simulink model "ver_602"  (R2015b)
settings: Solver=FixedStepDiscrete  StartTime=0.0  StopTime=inf  FixedStep=0.1  RelTol=1e-3
StartFcn:
  | %The GUI handles are by default hidden, turn them on
  | set(0,'ShowHiddenHandles','on');
  | 
  | %Set up the arguments that will go into the gain block event callback listener
  | blk = 'ver_601/Clock';
  | event = 'PostOutputs';
  | listener = @up_gui_ver_301;
  | 
  | %Create the listener
  | h = add_exec_event_listener(blk, event, listener);
settings Model: PauseTimes=26500  NumberOfSteps=10  Creator=Ridvan  LastModifiedBy=Edmem10

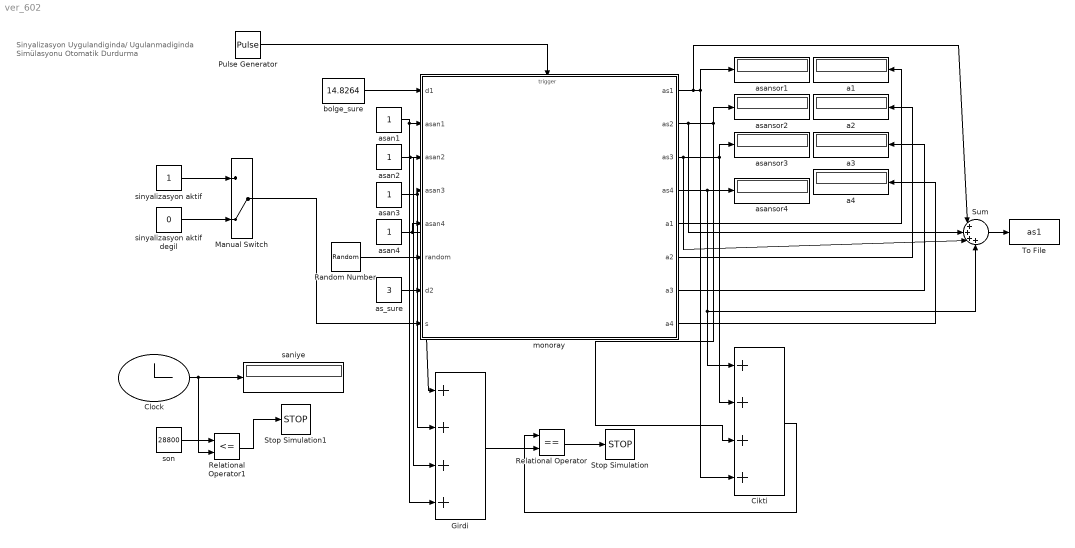
== system ver_602 ==
  note: Sinyalizasyon Uygulandiginda/ Ugulanmadiginda Simülasyonu Otomatik Durdurma
  Cikti : Sum  Inputs=++++
  Clock : Clock
      settings: Decimation=4
  Girdi : Sum  Inputs=++++
  Manual Switch : ManualSwitch  CurrentSetting=0
  Pulse Generator : DiscretePulseGenerator  PulseType=Time based  Period=1  PulseWidth=50
  Random Number : UniformRandomNumber  Minimum=0  Maximum=100  SampleTime=0.1
  Relational Operator : RelationalOperator  Operator===  OutDataTypeStr=boolean
  Relational Operator1 : RelationalOperator  Operator=<=  OutDataTypeStr=boolean
  Stop Simulation : Stop
  Stop Simulation1 : Stop
  Sum : Sum  Inputs=|++++
  To File : ToFile  Filename=as1  MatrixName=as1
  a{1..4} (4 alike) : Display
  as_sure : Constant  Value=3
  asan{1..4} (4 alike) : Constant
  asansor{1..4} (4 alike) : Display
  bolge_sure : Constant  Value=14.8264
  monoray : Stateflow chart  RequirementInfo="{}  %GIDa_5e52e2eb_da7a_4365_b597_b620b12073ae"  TreatAsAtomicUnit=on
  saniye : Display
  sinyalizasyon aktif : Constant
  sinyalizasyon aktif degil : Constant  Value=0
  son : Constant  Value=28800
  wires:
  Pulse Generator/1 -> monoray/Trigger
  monoray/2(as2) -> Sum/2, Cikti/3, asansor2/1
  monoray/1(as1) -> Sum/1, Cikti/4, asansor1/1
  monoray/3(as3) -> Sum/3, Cikti/2, asansor3/1
  bolge_sure/1 -> monoray/1(d1)
  Random Number/1 -> monoray/6(random)
  asan1/1 -> Girdi/4, monoray/2(asan1)
  asan2/1 -> Girdi/3, monoray/3(asan2)
  asan3/1 -> monoray/4(asan3), Girdi/2
  asan4/1 -> Girdi/1, monoray/5(asan4)
  as_sure/1 -> monoray/7(d2)
  monoray/5(a1) -> a1/1
  monoray/6(a2) -> a2/1
  monoray/7(a3) -> a3/1
  monoray/8(a4) -> a4/1
  Manual Switch/1 -> monoray/8(s)
  sinyalizasyon aktif/1 -> Manual Switch/1
  sinyalizasyon aktif degil/1 -> Manual Switch/2
  Clock/1 -> Relational Operator1/2, saniye/1
  Cikti/1 -> Relational Operator/1
  Girdi/1 -> Relational Operator/2
  Relational Operator/1 -> Stop Simulation/1
  Relational Operator1/1 -> Stop Simulation1/1
  son/1 -> Relational Operator1/1
  monoray/4(as4) -> Sum/4, Cikti/1, asansor4/1
  Sum/1 -> To File/1

== stateflow chart ver_602/monoray ==
  state m3
    state m1 [parallel]
      settings: executionOrder=1
      state r4 [parallel]
        settings: executionOrder=4
        state On
          en:vr4=1;
        state Next
          entry: vr5=1;
          dp5=dp4;
          vn5=vn4;
          vs5=vs4;
        state as1
          entry: as1 = as1 + 1;
          exit:dp4=0;
          vs4=0;
        state Off
          entry: vr4=0;
          dp4=0;
          vs4=0;
          vn4=0;
        m3.m1.r4.On -> m3.m1.r4.Next [order 2] : [after(d1, sec) & dp4~=1]
        m3.m1.r4.Off -> m3.m1.r4.On : [vr4==1]
        m3.m1.r4.On -> as1 [order 1] : [dp4==1 & after(d2,sec)]
        m3.m1.r4.Next -> m3.m1.r4.Off
        as1 -> m3.m1.r4.Next : [after(d1,sec)]{dp4=0;vs4=0;}
        (default) -> m3.m1.r4.Off
      state r5 [parallel]
        settings: executionOrder=5
        state On
          en:vr5=1;
        state Next1
          entry: vr6=1;
          dp6=dp5;
          vn6=vn5;
          vs6=vs5;
        state Next2
          entry: vr18=1;
          dp18=dp5;
          vn18=vn5;
          vs18=vs5;
        state Off
          entry: vr5=0;
          dp5=0;
          vs5=0;
          vn5=0;
        m3.m1.r5.On -> Next1 [order 2] : [after(d1, sec) & vr6==0]
        m3.m1.r5.On -> Next2 [order 1] : [(dp5==4 | dp5==0) & after(d1,sec) & vr18==0 & s==1]
        m3.m1.r5.Off -> m3.m1.r5.On : [vr5==1]
        Next1 -> m3.m1.r5.Off
        Next2 -> m3.m1.r5.Off
        (default) -> m3.m1.r5.Off
      state r8 [parallel]
        settings: executionOrder=8
        state On
          en:vr8=1;
        state Next
          entry: vr9=1;
          dp9=dp8;
          vn9=vn8;
          vs9=vs8;
        state Off
          entry: vr8=0;
          dp8=0;
          vs8=0;
          vn8=0;
        m3.m1.r8.On -> m3.m1.r8.Next : [after(d1, sec) & vr9==0]
        m3.m1.r8.Off -> m3.m1.r8.On : [vr8==1]
        m3.m1.r8.Next -> m3.m1.r8.Off
        (default) -> m3.m1.r8.Off
      state r9 [parallel]
        settings: executionOrder=9
        state On
          en:vr9=1;
        state Next
          entry: vr21=1;
          dp21=dp9;
          vn21=vn9;
          vs21=vs9;
        state Off
          entry: vr9=0;
          dp9=0;
          vs9=0;
          vn9=0;
        m3.m1.r9.On -> m3.m1.r9.Next : [after(d1, sec) & vr21==0]
        m3.m1.r9.Off -> m3.m1.r9.On : [vr9==1]
        m3.m1.r9.Next -> m3.m1.r9.Off
        (default) -> m3.m1.r9.Off
      state r6 [parallel]
        settings: executionOrder=6
        state On
          en:vr6=1;
        state Next
          entry: vr7=1;
          dp7=dp6;
          vn7=vn6;
          vs7=vs6;
        state Off
          entry: vr6=0;
          dp6=0;
          vs6=0;
          vn6=0;
        m3.m1.r6.On -> m3.m1.r6.Next : [after(d1, sec) & vr7==0]
        m3.m1.r6.Off -> m3.m1.r6.On : [vr6==1]
        m3.m1.r6.Next -> m3.m1.r6.Off
        (default) -> m3.m1.r6.Off
      state r7 [parallel]
        settings: executionOrder=7
        state On
          en:vr7=1;
        state Next
          entry: vr8=1;
          dp8=dp7;
          vn8=vn7;
          vs8=vs7;
        state as2
          entry: as2 = as2 + 1;
          exit: dp7=0;
          vs7=0;
        state Off
          entry: vr7=0;
          dp7=0;
          vs7=0;
          vn7=0;
        m3.m1.r7.On -> m3.m1.r7.Next [order 2] : [after(d1, sec) & vr8==0 ]
        m3.m1.r7.On -> as2 [order 1] : [dp7==2&after(d2,sec)]
        m3.m1.r7.Off -> m3.m1.r7.On : [vr7==1]
        as2 -> m3.m1.r7.Next : [after(d1,sec)]{dp7=0;vs7=0;}
        m3.m1.r7.Next -> m3.m1.r7.Off
        (default) -> m3.m1.r7.Off
      state r3 [parallel]
        settings: executionOrder=3
        state On
          en:vr3=1;
        state Next
          entry: vr24=1;
          dp24=dp3;
          vn24=vn3;
          vs24=vs3;
        state Off
          entry: vr3=0;
          dp3=0;
          vs3=0;
          vn3=0;
        m3.m1.r3.On -> m3.m1.r3.Next : [after(d1, sec) & vr24==0]
        m3.m1.r3.Off -> m3.m1.r3.On : [vr3==1]
        (default) -> m3.m1.r3.Off
        m3.m1.r3.Next -> m3.m1.r3.Off
      state r20 [parallel]
        settings: executionOrder=18
        state On
          en:vr20=1;
        state Next
          entry: vr4=1;
          dp4=dp20;
          vn4=vn20;
          vs4=vs20;
        state Off
          entry: vr20=0;
          dp20=0;
          vs20=0;
          vn20=0;
        m3.m1.r20.On -> m3.m1.r20.Next : [after(d1, sec) & vr4==0]
        m3.m1.r20.Off -> m3.m1.r20.On : [vr20==1]
        (default) -> m3.m1.r20.Off
        m3.m1.r20.Next -> m3.m1.r20.Off
      state r24 [parallel]
        settings: executionOrder=21
        state On
          en:vr24=1;
        state Next
          entry: vr20=1;
          dp20=dp24;
          vn20=vn24;
          vs20=vs24;
        state Off
          entry: vr24=0;
          dp24=0;
          vs24=0;
          vn24=0;
        m3.m1.r24.On -> m3.m1.r24.Next : [after(d1, sec) & vr20==0]
        m3.m1.r24.Off -> m3.m1.r24.On : [vr24==1]
        m3.m1.r24.Next -> m3.m1.r24.Off
        (default) -> m3.m1.r24.Off
      state tictoc [parallel]
        settings: executionOrder=26
        state tic
        state toc
        (default) -> tic
        tic -> toc : {color1}
        toc -> tic
      state r2 [parallel]
        settings: executionOrder=2
        state On
          en:vr2=1;
        state Next
          entry: vr3=1;
          dp3=dp2;
          vn3=vn2;
          vs3=vs2;
        state Off
          entry: vr2=0;
          dp2=0;
          vs2=0;
          vn2=0;
        m3.m1.r2.On -> m3.m1.r2.Next : [after(d1, sec) & vr3==0]
        m3.m1.r2.Off -> m3.m1.r2.On : [vr2==1]
        m3.m1.r2.Next -> m3.m1.r2.Off
        (default) -> m3.m1.r2.Off
      state r21 [parallel]
        settings: executionOrder=19
        state On
          en:vr21=1;
        state Next
          entry: vr22=1;
          dp22=dp21;
          vn22=vn21;
          vs22=vs21;
        state Off
          entry: vr21=0;
          dp21=0;
          vs21=0;
          vn21=0;
        m3.m1.r21.On -> m3.m1.r21.Next : [after(d1, sec) & vr22==0]
        m3.m1.r21.Off -> m3.m1.r21.On : [vr21==1]
        m3.m1.r21.Next -> m3.m1.r21.Off
        (default) -> m3.m1.r21.Off
      state r18 [parallel]
        settings: executionOrder=16
        state On
          en:vr18=1;
        state Next
          entry: vr14=1;
          dp14=dp18;
          vn14=vn18;
          vs14=vs18;
        state Off
          entry: vr18=0;
          dp18=0;
          vs18=0;
          vn18=0;
        m3.m1.r18.On -> m3.m1.r18.Next : [after(d1, sec) & vr14==0 & vr13==0]
        m3.m1.r18.Off -> m3.m1.r18.On : [vr18==1]
        m3.m1.r18.Next -> m3.m1.r18.Off
        (default) -> m3.m1.r18.Off
      state r1 [parallel]
        settings: executionOrder=1
        state On
          en:vr1=1;
        state Next
          entry: vr19=1;
          dp19=j1;
          vs19=1;
        state Off
          entry: vr1=0;
          dp1=0;
          vs1=0;
        m3.m1.r1.On -> m3.m1.r1.Next : [j1>0 & vr19==1 & vs19==0 & after((d1+d2),sec) ]
        m3.m1.r1.Off -> m3.m1.r1.On : [ j1>0]
        m3.m1.r1.Next -> m3.m1.r1.Off
        (default) -> m3.m1.r1.Off
      state r19 [parallel]
        settings: executionOrder=17
        state On
          en:vr19=1;
        state Next
          entry: vr2=1;
          dp2=dp19;
          vn2=vn19;
          vs2=vs19;
          vn19=0;
        state Off
          entry: vr19=0;
          dp19=0;
          vs19=0;
        (default) -> m3.m1.r19.On : {vn19=1;vs19=0;}
        m3.m1.r19.On -> m3.m1.r19.Next : [after(d2, sec) & vr2==0 & vs19>0]
        m3.m1.r19.Off -> m3.m1.r19.On : [vr19==1]
        m3.m1.r19.Next -> m3.m1.r19.Off
      state r22 [parallel]
        settings: executionOrder=20
        state On
          en:vr22=1;
        state Next
          entry: vr10=1;
          dp10=dp22;
          vn10=vn22;
          vs10=vs22;
        state Off
          entry: vr22=0;
          dp22=0;
          vs22=0;
          vn22=0;
        m3.m1.r22.On -> m3.m1.r22.Next : [after(d1, sec) & vr10==0]
        m3.m1.r22.Off -> m3.m1.r22.On : [vr22==1]
        m3.m1.r22.Next -> m3.m1.r22.Off
        (default) -> m3.m1.r22.Off
      state r17 [parallel]
        settings: executionOrder=15
        state On
          en:vr17=1;
        state Next
          entry: vr19=1;
          dp19=dp17;
          vn19=vn17;
          vs19=vs17;
        state Off
          entry: vr17=0;
          dp17=0;
          vs17=0;
          vn17=0;
        (default) -> m3.m1.r17.On : {vn17=2;vs17=0;dp17=0;}
        m3.m1.r17.On -> m3.m1.r17.Next : [after(d1, sec) & vr19==0]
        m3.m1.r17.Off -> m3.m1.r17.On : [vr17==1]
        m3.m1.r17.Next -> m3.m1.r17.Off
      state r12 [parallel]
        settings: executionOrder=12
        state On
          en:vr12=1;
        state Next
          entry: vr13=1;
          dp13=dp12;
          vn13=vn12;
          vs13=vs12;
        state as3
          entry: as3 = as3 + 1;
          exit:dp12=0;
          vs12=0;
        state Off
          entry: vr12=0;
          dp12=0;
          vs12=0;
          vn12=0;
        m3.m1.r12.On -> m3.m1.r12.Next [order 2] : [after(d1, sec) & vr13==0 ]
        m3.m1.r12.Off -> m3.m1.r12.On : [vr12==1]
        m3.m1.r12.On -> as3 [order 1] : [dp12==3&after(d2,sec)]
        as3 -> m3.m1.r12.Next : [after(d1,sec)]{dp12=0;vs12=0;}
        m3.m1.r12.Next -> m3.m1.r12.Off
        (default) -> m3.m1.r12.Off
      state r15 [parallel]
        settings: executionOrder=22
        state On
          en:vr15=1;
        state Next
          entry: vr25=1;
          dp25=dp15;
          vn25=vn15;
          vs25=vs15;
        state Off
          entry: vr15=0;
          dp15=0;
          vs15=0;
          vn15=0;
        state as4
          entry: as4 = as4 + 1;
          exit: dp15=0;
          vs15=0;
        m3.m1.r15.On -> as4 [order 1] : [dp15==4&after(d2,sec)]
        m3.m1.r15.On -> m3.m1.r15.Next [order 2] : [after(d1, sec) & vr25==0]
        m3.m1.r15.Off -> m3.m1.r15.On : [vr15==1]
        m3.m1.r15.Next -> m3.m1.r15.Off
        as4 -> m3.m1.r15.Next : [after(d1,sec)]{dp15=0;vs15=0;}
        (default) -> m3.m1.r15.Off
      state r14 [parallel]
        settings: executionOrder=14
        state On
          en:vr14=1;
        state Next
          entry: vr15=1;
          dp15=dp14;
          vn15=vn14;
          vs15=vs14;
        state Off
          entry: vr14=0;
          dp14=0;
          vs14=0;
          vn14=0;
        m3.m1.r14.On -> m3.m1.r14.Next : [after(d1, sec) & vr15==0]
        m3.m1.r14.Off -> m3.m1.r14.On : [vr14==1]
        m3.m1.r14.Next -> m3.m1.r14.Off
        (default) -> m3.m1.r14.Off
      state r10 [parallel]
        settings: executionOrder=10
        state On
          en:vr10=1;
        state Next
          entry: vr11=1;
          dp11=dp10;
          vn11=vn10;
          vs11=vs10;
        state Off
          entry: vr10=0;
          dp10=0;
          vs10=0;
        m3.m1.r10.On -> m3.m1.r10.Next : [after(d1, sec) & vr11==0]
        m3.m1.r10.Off -> m3.m1.r10.On : [vr10==1]
        m3.m1.r10.Next -> m3.m1.r10.Off
        (default) -> m3.m1.r10.Off
      state r11 [parallel]
        settings: executionOrder=11
        state On
          en:vr11=1;
        state Next
          entry: vr12=1;
          dp12=dp11;
          vn12=vn11;
          vs12=vs11;
        state Off
          entry: vr11=0;
          dp11=0;
          vs11=0;
          vn11=0;
        m3.m1.r11.On -> m3.m1.r11.Next : [after(d1, sec) & vr12==0]
        m3.m1.r11.Off -> m3.m1.r11.On : [vr11==1]
        m3.m1.r11.Next -> m3.m1.r11.Off
        (default) -> m3.m1.r11.Off
      state r16 [parallel]
        settings: executionOrder=23
        state On
          en:vr16=1;
        state Off
          entry: vr16=0;
          dp16=0;
          vs16=0;
          vn16=0;
        state Next
          entry: vr17=1;
          dp17=dp16;
          vn17=vn16;
          vs17=vs16;
        (default) -> m3.m1.r16.On : {vn16=3;vs16=0;dp16=0;}
        m3.m1.r16.On -> m3.m1.r16.Next : [after(d1,sec) & vr17==0]
        m3.m1.r16.Off -> m3.m1.r16.On : [vr16==1]
        m3.m1.r16.Next -> m3.m1.r16.Off
      state r23 [parallel]
        settings: executionOrder=24
        state On
          en:vr23=1;
        state Next
          entry: vr16=1;
          dp16=dp23;
          vn16=vn23;
          vs16=vs23;
        state Off
          entry: vr23=0;
          dp23=0;
          vs23=0;
          vn23=0;
        (default) -> m3.m1.r23.On : {vn23=4;vs23=0;dp23=0;}
        m3.m1.r23.On -> m3.m1.r23.Next : [after(d1,sec) & vr16==0]
        m3.m1.r23.Off -> m3.m1.r23.On : [vr23==1]
        m3.m1.r23.Next -> m3.m1.r23.Off
      state r13 [parallel]
        settings: executionOrder=13
        state On
          en:vr13=1;
        state Next
          entry: vr14=1;
          dp14=dp13;
          vn14=vn13;
          vs14=vs13;
        state Off
          entry: vr13=0;
          dp13=0;
          vs13=0;
          vn13=0;
        m3.m1.r13.On -> m3.m1.r13.Next : [ vr14==0 &after(d1, sec)]
        m3.m1.r13.Off -> m3.m1.r13.On : [vr13==1]
        m3.m1.r13.Next -> m3.m1.r13.Off
        (default) -> m3.m1.r13.Off
      state r25 [parallel]
        settings: executionOrder=25
        state On
          en:vr25=1;
        state Next
          entry: vr23=1;
          dp23=dp25;
          vn23=vn25;
          vs23=vs25;
        state Off
          entry: vr25=0;
          dp25=0;
          vs25=0;
          vn25=0;
        m3.m1.r25.On -> m3.m1.r25.Next : [after(d1,sec) & vr23==0]
        m3.m1.r25.Off -> m3.m1.r25.On : [vr25==1]
        m3.m1.r25.Next -> m3.m1.r25.Off
        (default) -> m3.m1.r25.Off
    state rdn [parallel]
      settings: executionOrder=2
      state rndm
      state job_0
        entry: j1=0;
      state job_04
        entry: j1=4;
        exit:a4 = a4 - 1;
      state job_01
        entry: j1=1;
        exit:a1 = a1 - 1;
      state job_03
        entry: j1=3;
        exit:a3 = a3 - 1;
      state job_02
        entry: j1=2;
        exit:a2 = a2 - 1;
      (default) -> rndm : {a1=asan1;a2=asan2;a3=asan3;a4=asan4;}
      job_0 -> rndm
      rndm -> (junction 382) : [vr19==1]
      (junction 358) -> rndm : [vr19==0]
      (junction 382) -> job_0 [order 5] : [a1==0 | a2==0 | a3==0 | a4==0]
      job_04 -> (junction 358)
      (junction 382) -> job_04 [order 1] : [a4>0&(75<= random)]
      (junction 382) -> job_01 [order 4] : [a1>0&(0<= random) & (random<25)]
      (junction 382) -> job_02 [order 3] : [a2>0&(25<=random) & (random<50)]
      (junction 382) -> job_03 [order 2] : [a3>0&(50<=random) & (random<75)]
      job_01 -> (junction 358)
      job_03 -> (junction 358)
      job_02 -> (junction 358)
  data: vr1 local =0; vr2 local =0; j1 local [0..2] =0; vr7 local; vr6 local; vr8 local; vr5 local; vr3 local =0; vr4 local; as1 output =0; vr9 local; vr11 local; vr12 local; vr10 local =0; as2 output =0; vr17 local =0; vr13 local =0; as3 output =0; vr14 local =0; vr15 local =0; vr16 local =0; as4 output =0; a1 output; a2 output; a3 output; d1 input; vr18 local; vr19 local =0; vs3 local; vn3 local; dp3 local; vn19 local; vs19 local; dp19 local =0; dp2 local; vn2 local; vs2 local; dp1 local; vs1 local; vn7 local; vs7 local; dp10 local; vn10 local; vs10 local; dp11 local; vn11 local; dp16 local; dp13 local; dp12 local; vn15 local; vn16 local; dp15 local; vs14 local; vn14 local; dp14 local; vs17 local; vs12 local; vs13 local; vn12 local; vn17 local; dp17 local; vs11 local; vs16 local; vs15 local; vn13 local; dp4 local; vn4 local; vs4 local; dp5 local; vn5 local; vs5 local; dp6 local; vn6 local; vs6 local; dp18 local; vn18 local; vs18 local; dp9 local; dp8 local; vn9 local; vn8 local; vs9 local; vs8 local; dp7 local; vr22 local; dp22 local; vn22 local; vs22 local; vs23 local; vr23 local; dp23 local; vn23 local; vs21 local; vr21 local; dp21 local; vn21 local; vr20 local; dp20 local; vn20 local; vs20 local; asan1 input; asan2 input; asan3 input; asan4 input; a4 output; random input; d2 input; vr25 local; vs25 local; vn25 local; dp25 local; dp24 local; vn24 local; vr24 local; vs24 local; s input
  events: trig input RISING_EDGE_EVENT
  function color1:
    | function color1
    | 
    | txt1 = findobj('Tag','text_vr1');
    | txt19 = findobj('Tag','text_vr19');
    | txt2 = findobj('Tag','text_vr2');
    | txt3 = findobj('Tag','text_vr3');
    | txt24 = findobj('Tag','text_vr24');
    | txt20 = findobj('Tag','text_vr20');
    | txt4 = findobj('Tag','text_vr4');
    | txt5 = findobj('Tag','text_vr5');
    | txt18 = findobj('Tag','text_vr18');
    | txt6 = findobj('Tag','text_vr6');
    | txt7 = findobj('Tag','text_vr7');
    | txt8 = findobj('Tag','text_vr8');
    | txt9 = findobj('Tag','text_vr9');
    | txt21 = findobj('Tag','text_vr21');
    | txt22 = findobj('Tag','text_vr22');
    | txt10 = findobj('Tag','text_vr10');
    | txt11 = findobj('Tag','text_vr11');
    | txt12 = findobj('Tag','text_vr12');
    | txt13 = findobj('Tag','text_vr13');
    | txt14 = findobj('Tag','text_vr14');
    | txt15 = findobj('Tag','text_vr15');
    | txt25 = findobj('Tag','text_vr25');
    | txt23 = findobj('Tag','text_vr23');
    | txt16 = findobj('Tag','text_vr16');
    | txt17 = findobj('Tag','text_vr17');
    | 
    | txt_as1 = findobj('Tag','text_as1');
    | txt_as2 = findobj('Tag','text_as2');
    | txt_as3 = findobj('Tag','text_as3');
    | txt_as4 = findobj('Tag','text_as4');
    | 
    | edt_as1 = findobj('Tag','edit_as1');
    | set(edt_as1,'String',as1);
    | edt_as2 = findobj('Tag','edit_as2');
    | set(edt_as2,'String',as2);
    | edt_as3 = findobj('Tag','edit_as3');
    | set(edt_as3,'String',as3);
    | edt_as4 = findobj('Tag','edit_as4');
    | set(edt_as4,'String',as4);
    | 
    | if vr1==1
    | set(txt1,'BackgroundColor','green');
    | else
    | set(txt1,'BackgroundColor','white'); 
    | end
    | 
    | if vr2==1
    | set(txt2,'BackgroundColor','green');
    | set(txt2,'String',[vn2 dp2]);
    | else
    | set(txt2,'BackgroundColor','white');
    | set(txt2,'String','');
    | end
    | 
    | if vr3==1
    | set(txt3,'BackgroundColor','green');
    | set(txt3,'String',[vn3 dp3]);
    | else
    | set(txt3,'BackgroundColor','white');
    | set(txt3,'String','');
    | end
    | 
    | if vr4==1
    | set(txt4,'BackgroundColor','green');
    | set(txt4,'String',[vn4 dp4]);
    | else
    | set(txt4,'BackgroundColor','white');
    | set(txt4,'String','');
    | end
    | 
    | if vr5==1
    | set(txt5,'BackgroundColor','green');
    | set(txt5,'String',[vn5 dp5]);
    | else
    | set(txt5,'BackgroundColor','white');
    | set(txt5,'String','');
    | end
    | 
    | if vr6==1
    | set(txt6,'BackgroundColor','green');
    | set(txt6,'String',[vn6 dp6]);
    | else
    | set(txt6,'BackgroundColor','white'); 
    | set(txt6,'String','');
    | end
    | 
    |   if vr7==1
    | set(txt7,'BackgroundColor','green');
    | set(txt7,'String',[vn7 dp7]);
    |   else
    | set(txt7,'BackgroundColor','white');
    | set(txt7,'String','');
    |   end
    | 
    |   if vr8==1
    | set(txt8,'BackgroundColor','green');
    | set(txt8,'String',[vn8 dp8]);
    |   else
    | set(txt8,'BackgroundColor','white');
    | set(txt8,'String','');
    |   end
    |   
    |   if vr9==1
    | set(txt9,'BackgroundColor','green');
    | set(txt9,'String',[vn9 dp9]);
    |   else
    | set(txt9,'BackgroundColor','white');
    | set(txt9,'String','');
    |   end
    | 
    |   if vr10==1
    | set(txt10,'BackgroundColor','green');
    | set(txt10,'String',[vn10 dp10]);
    |   else
    | set(txt10,'BackgroundColor','white');
    | set(txt10,'String','');
    |   end
    |   if vr11==1
    | set(txt11,'BackgroundColor','green');
    | set(txt11,'String',[vn11 dp11]);
    |   else
    | set(txt11,'BackgroundColor','white');
    | set(txt11,'String','');
    |   end
    |   if vr12==1
    | set(txt12,'BackgroundColor','green');
    | set(txt12,'String',[vn12 dp12]);
    |   else
    | set(txt12,'BackgroundColor','white');
    | set(txt12,'String','');
    |   end
    |   if vr13==1
    | set(txt13,'BackgroundColor','green');
    | set(txt13,'String',[vn13 dp13]);
    |   else
    | set(txt13,'BackgroundColor','white');
    | set(txt13,'String','');
    |   end
    |   if vr14==1
    | set(txt14,'BackgroundColor','green');
    | set(txt14,'String',[vn14 dp14]);
    |   else
    | set(txt14,'BackgroundColor','white');
    | set(txt14,'String','');
    |   end
    |   if vr15==1
    | set(txt15,'BackgroundColor','green');
    | set(txt15,'String',[vn15 dp15]);
    |   else
    | set(txt15,'BackgroundColor','white');
    | set(txt15,'String','');
    |   end
    |   if vr16==1
    | set(txt16,'BackgroundColor','green');
    | set(txt16,'String',[vn16 dp16]);
    |   else
    | set(txt16,'BackgroundColor','white');
    | set(txt16,'String','');
    |   end
    |   if vr17==1
    | set(txt17,'BackgroundColor','green');
    | set(txt17,'String',[vn17 dp17]);
    |   else
    | set(txt17,'BackgroundColor','white');
    | set(txt17,'String','');
    |   end
    |   if vr18==1
    | set(txt18,'BackgroundColor','green');
    | set(txt18,'String',[vn18 dp18]);
    |   else
    | set(txt18,'BackgroundColor','white');
    | set(txt18,'String','');
    |   end
    |   if vr19==1
    | set(txt19,'BackgroundColor','green');
    | set(txt19,'String',[vn19 dp19]);
    |   else
    | set(txt19,'BackgroundColor','white');
    | set(txt19,'String','');
    |   end
    |   if vr20==1
    | set(txt20,'BackgroundColor','green');
    | set(txt20,'String',[vn20 dp20]);
    |   else
    | set(txt20,'BackgroundColor','white');
    | set(txt20,'String','');
    |   end
    |   if vr21==1
    | set(txt21,'BackgroundColor','green');
    | set(txt21,'String',[vn21 dp21]);
    |   else
    | set(txt21,'BackgroundColor','white');
    | set(txt21,'String','');
    |   end
    |   if vr22==1
    | set(txt22,'BackgroundColor','green');
    | set(txt22,'String',[vn22 dp22]);
    |   else
    | set(txt22,'BackgroundColor','white');
    | set(txt22,'String','');
    |   end
    |   if vr23==1
    | set(txt23,'BackgroundColor','green');
    | set(txt23,'String',[vn23 dp23]);
    |   else
    | set(txt23,'BackgroundColor','white');
    | set(txt23,'String','');
    |   end
    |   if vr24==1
    | set(txt24,'BackgroundColor','green');
    | set(txt24,'String',[vn24 dp24]);
    |   else
    | set(txt24,'BackgroundColor','white');
    | set(txt24,'String','');
    |   end
    |   if vr25==1
    | set(txt25,'BackgroundColor','green');
    | set(txt25,'String',[vn25 dp25]);
    |   else
    | set(txt25,'BackgroundColor','white');
    | set(txt25,'String','');
    |   end
    |  
    |  if dp4==1
    | set(txt_as1,'BackgroundColor','yellow');
    |   else
    | set(txt_as1,'BackgroundColor','white');
    |  end
    |  
    |    if dp7==2
    | set(txt_as2,'BackgroundColor','yellow');
    |   else
    | set(txt_as2,'BackgroundColor','white');
    |    end
    |    
    |    if dp12==3
    | set(txt_as3,'BackgroundColor','yellow');
    |   else
    | set(txt_as3,'BackgroundColor','white');
    |    end
    |    
    |    if dp15==4
    | set(txt_as4,'BackgroundColor','yellow');
    |   else
    | set(txt_as4,'BackgroundColor','white');
    |   end
